simulink model "snb_bx"  (R2012b)
settings: Solver=FixedStepDiscrete  SolverMode=SingleTasking  StartTime=0.0  StopTime=10000  RelTol=1e-3
undefined symbols (not defined in the file): Down, pfb_coeff_gen_calc, Up, xlipgetpartsetting
libraries: xbsIndex_r4 x14917, casper_library_misc x20, casper_library_communications x8, xps_library x3, casper_library_delays x3
(part 48 of 96)

== system snb_bx/mix_dec_fir/dec_fir_async/fir_col_async3 ==
  dbus_in : Inport
  dbus_back_in : Inport  Port=2
  dv : Inport  Port=3
  adder_tree1 : Subsystem  AncestorBlock=casper_library_misc/adder_tree  mask(adder_tree){n_inputs=8, latency=3, adder_imp=Behavioral, first_stage_hdl=off}
      mask prompts: n_inputs "Number of Inputs"; latency "Add Latency"; adder_imp "Adder implementation"; first_stage_hdl "Use behavioural HDL for first stage of adders"
      mask help:
      | Sums all inputs using a tree of adds and delays.
      |
      | Number of inputs: The number of inputs to the block to be summed
      | Add latency: The number of clock cycles to perform one addition (affects timing)..
      | Adder implementation: choice of fabric or DSP48E core, or behavioral HDL
      | Use behavioural HDL for first stage of adders: Causes the first stage of adders to be absorbed into DSP blocks if multipliers precede them (Virtex 5). Overrides Adder implementation
      mask init:
      | adder_tree_init(gcb, ...
      |     'n_inputs', n_inputs, ...
      |     'latency', latency, ...
      |     'adder_imp', adder_imp, ...
      |     'first_stage_hdl', first_stage_hdl);
      settings: AttributesFormatString=latency 9
      mask Help: eval('xlWeb(''http://casper.berkeley.edu/wiki/Adder_tree'')')
      mask TypeOptions adder_imp: Behavioral | Fabric | DSP48
  adder_tree2 : Subsystem  AncestorBlock=casper_library_misc/adder_tree  mask(adder_tree){n_inputs=8, latency=3, adder_imp=Behavioral, first_stage_hdl=off}
      mask prompts: n_inputs "Number of Inputs"; latency "Add Latency"; adder_imp "Adder implementation"; first_stage_hdl "Use behavioural HDL for first stage of adders"
      mask help:
      | Sums all inputs using a tree of adds and delays.
      |
      | Number of inputs: The number of inputs to the block to be summed
      | Add latency: The number of clock cycles to perform one addition (affects timing)..
      | Adder implementation: choice of fabric or DSP48E core, or behavioral HDL
      | Use behavioural HDL for first stage of adders: Causes the first stage of adders to be absorbed into DSP blocks if multipliers precede them (Virtex 5). Overrides Adder implementation
      mask init:
      | adder_tree_init(gcb, ...
      |     'n_inputs', n_inputs, ...
      |     'latency', latency, ...
      |     'adder_imp', adder_imp, ...
      |     'first_stage_hdl', first_stage_hdl);
      settings: AttributesFormatString=latency 9
      mask Help: eval('xlWeb(''http://casper.berkeley.edu/wiki/Adder_tree'')')
      mask TypeOptions adder_imp: Behavioral | Fabric | DSP48
  c1 : xbsIndex_r4/Constant  const=1  gui_display_data_type=Fixed-point  arith_type=Signed (2's comp)  n_bits=16  bin_pt=14  preci_type=Single  exp_width=8  frac_width=24  explicit_period=on  period=1  equ=P=C  opselect=C  inp2=PCIN>>17  opr=+  inp1=P  carry=CIN  dbl_ovrd=off  block_type=constant
  c2 : xbsIndex_r4/Constant  const=1  gui_display_data_type=Fixed-point  arith_type=Signed (2's comp)  n_bits=16  bin_pt=14  preci_type=Single  exp_width=8  frac_width=24  explicit_period=on  period=1  equ=P=C  opselect=C  inp2=PCIN>>17  opr=+  inp1=P  carry=CIN  dbl_ovrd=off  block_type=constant
  fir_tap1 : Subsystem  AncestorBlock=casper_library_downconverter/fir_tap_async  mask(fir_tap_async){factor=0.028683, add_latency=3, mult_latency=2, coeff_bit_width=24, coeff_bin_pt=23, async=on, dbl=on}
      mask prompts: add_latency "Add latency"; mult_latency "Mult latency"; coeff_bit_width "Coefficient bit width"; coeff_bin_pt "Coefficient binary point"; async "Asynchronous ops"; dbl "Double tap"
      mask help: Multiplies input data with factor specified.
      mask init:
      | fir_tap_async_init(gcb);
      mask Help: eval('xlWeb(''http://casper.berkeley.edu/wiki/Fir_tap'')')
  fir_tap2 : Subsystem  AncestorBlock=casper_library_downconverter/fir_tap_async  mask(fir_tap_async){factor=0.026325, add_latency=3, mult_latency=2, coeff_bit_width=24, coeff_bin_pt=23, async=on, dbl=on}
      mask prompts: add_latency "Add latency"; mult_latency "Mult latency"; coeff_bit_width "Coefficient bit width"; coeff_bin_pt "Coefficient binary point"; async "Asynchronous ops"; dbl "Double tap"
      mask help: Multiplies input data with factor specified.
      mask init:
      | fir_tap_async_init(gcb);
      mask Help: eval('xlWeb(''http://casper.berkeley.edu/wiki/Fir_tap'')')
  fir_tap3 : Subsystem  AncestorBlock=casper_library_downconverter/fir_tap_async  mask(fir_tap_async){factor=0.023903, add_latency=3, mult_latency=2, coeff_bit_width=24, coeff_bin_pt=23, async=on, dbl=on}
      mask prompts: add_latency "Add latency"; mult_latency "Mult latency"; coeff_bit_width "Coefficient bit width"; coeff_bin_pt "Coefficient binary point"; async "Asynchronous ops"; dbl "Double tap"
      mask help: Multiplies input data with factor specified.
      mask init:
      | fir_tap_async_init(gcb);
      mask Help: eval('xlWeb(''http://casper.berkeley.edu/wiki/Fir_tap'')')
  fir_tap4 : Subsystem  AncestorBlock=casper_library_downconverter/fir_tap_async  mask(fir_tap_async){factor=0.021464, add_latency=3, mult_latency=2, coeff_bit_width=24, coeff_bin_pt=23, async=on, dbl=on}
      mask prompts: add_latency "Add latency"; mult_latency "Mult latency"; coeff_bit_width "Coefficient bit width"; coeff_bin_pt "Coefficient binary point"; async "Asynchronous ops"; dbl "Double tap"
      mask help: Multiplies input data with factor specified.
      mask init:
      | fir_tap_async_init(gcb);
      mask Help: eval('xlWeb(''http://casper.berkeley.edu/wiki/Fir_tap'')')
  fir_tap5 : Subsystem  AncestorBlock=casper_library_downconverter/fir_tap_async  mask(fir_tap_async){factor=0.01905, add_latency=3, mult_latency=2, coeff_bit_width=24, coeff_bin_pt=23, async=on, dbl=on}
      mask prompts: add_latency "Add latency"; mult_latency "Mult latency"; coeff_bit_width "Coefficient bit width"; coeff_bin_pt "Coefficient binary point"; async "Asynchronous ops"; dbl "Double tap"
      mask help: Multiplies input data with factor specified.
      mask init:
      | fir_tap_async_init(gcb);
      mask Help: eval('xlWeb(''http://casper.berkeley.edu/wiki/Fir_tap'')')
  fir_tap6 : Subsystem  AncestorBlock=casper_library_downconverter/fir_tap_async  mask(fir_tap_async){factor=0.016702, add_latency=3, mult_latency=2, coeff_bit_width=24, coeff_bin_pt=23, async=on, dbl=on}
      mask prompts: add_latency "Add latency"; mult_latency "Mult latency"; coeff_bit_width "Coefficient bit width"; coeff_bin_pt "Coefficient binary point"; async "Asynchronous ops"; dbl "Double tap"
      mask help: Multiplies input data with factor specified.
      mask init:
      | fir_tap_async_init(gcb);
      mask Help: eval('xlWeb(''http://casper.berkeley.edu/wiki/Fir_tap'')')
  fir_tap7 : Subsystem  AncestorBlock=casper_library_downconverter/fir_tap_async  mask(fir_tap_async){factor=0.014454, add_latency=3, mult_latency=2, coeff_bit_width=24, coeff_bin_pt=23, async=on, dbl=on}
      mask prompts: add_latency "Add latency"; mult_latency "Mult latency"; coeff_bit_width "Coefficient bit width"; coeff_bin_pt "Coefficient binary point"; async "Asynchronous ops"; dbl "Double tap"
      mask help: Multiplies input data with factor specified.
      mask init:
      | fir_tap_async_init(gcb);
      mask Help: eval('xlWeb(''http://casper.berkeley.edu/wiki/Fir_tap'')')
  fir_tap8 : Subsystem  AncestorBlock=casper_library_downconverter/fir_tap_async  mask(fir_tap_async){factor=0.012336, add_latency=3, mult_latency=2, coeff_bit_width=24, coeff_bin_pt=23, async=on, dbl=on}
      mask prompts: add_latency "Add latency"; mult_latency "Mult latency"; coeff_bit_width "Coefficient bit width"; coeff_bin_pt "Coefficient binary point"; async "Asynchronous ops"; dbl "Double tap"
      mask help: Multiplies input data with factor specified.
      mask init:
      | fir_tap_async_init(gcb);
      mask Help: eval('xlWeb(''http://casper.berkeley.edu/wiki/Fir_tap'')')
  inbus : Subsystem  AncestorBlock=casper_library_flow_control/bus_expand  mask(bus_expand){mode=divisions of equal size, outputNum=16, outputWidth=20, outputBinaryPt=18, outputArithmeticType=1, show_format=off, outputToWorkspace=off, variablePrefix=out, outputToModelAsWell=on}
      mask prompts: outputNum "Number of outputs:"; outputWidth "Output width:"; outputBinaryPt "Output binary point position:"; outputArithmeticType "Output arithmetic type (ufix=0, fix=1, bool=2):"; show_format "Print format string?"; outputToWorkspace "Output to workspace?"; variablePrefix "Variable name prefix:"; outputToModelAsWell "Output to model as well?"
      mask help:
      | Expands a 'bus' made using a bus_create or Xilinx
      | concat block.
      | The input will be divided into the specified number
      | of outputs with the specified arithmetic types.
      | Divisions are made from most significant bit.
      mask init: same as snb_bx/bus_expand10
      settings: AttributesFormatString=16 outputs
      mask TypeOptions mode: divisions of equal size | divisions of arbitrary size
      mask Callback mode: bus_expand_callback();
      mask Callback outputWidth: bus_expand_callback();
      mask Callback outputToWorkspace: bus_expand_callback();
  inbus_back : Subsystem  AncestorBlock=casper_library_flow_control/bus_expand  mask(bus_expand){mode=divisions of equal size, outputNum=16, outputWidth=20, outputBinaryPt=18, outputArithmeticType=1, show_format=off, outputToWorkspace=off, variablePrefix=out, outputToModelAsWell=on}
      mask prompts: outputNum "Number of outputs:"; outputWidth "Output width:"; outputBinaryPt "Output binary point position:"; outputArithmeticType "Output arithmetic type (ufix=0, fix=1, bool=2):"; show_format "Print format string?"; outputToWorkspace "Output to workspace?"; variablePrefix "Variable name prefix:"; outputToModelAsWell "Output to model as well?"
      mask help:
      | Expands a 'bus' made using a bus_create or Xilinx
      | concat block.
      | The input will be divided into the specified number
      | of outputs with the specified arithmetic types.
      | Divisions are made from most significant bit.
      mask init: same as snb_bx/bus_expand10
      settings: AttributesFormatString=16 outputs
      mask TypeOptions mode: divisions of equal size | divisions of arbitrary size
      mask Callback mode: bus_expand_callback();
      mask Callback outputWidth: bus_expand_callback();
      mask Callback outputToWorkspace: bus_expand_callback();
  outbus : Subsystem  AncestorBlock=casper_library_flow_control/bus_create  mask(bus_create){inputNum=16}
      mask prompts: inputNum "Number of inputs:"
      mask init:
      | bus_create_init(gcb,...
      |     'inputNum', inputNum);
  outbus_back : Subsystem  AncestorBlock=casper_library_flow_control/bus_create  mask(bus_create){inputNum=16}
      mask prompts: inputNum "Number of inputs:"
      mask init:
      | bus_create_init(gcb,...
      |     'inputNum', inputNum);
  term1 : Terminator
  term2 : Terminator
  dbus_out : Outport
  dbus_back_out : Outport  Port=2
  real_sum : Outport  Port=3
  imag_sum : Outport  Port=4
  wires:
  dbus_in/1 -> inbus/1(bus_in)
  dbus_back_in/1 -> inbus_back/1(bus_in)
  dv/1 -> [dv_in]
  [dv_in] -> fir_tap1/5(dv_in)
  inbus/1(msb_out16) -> fir_tap1/1(a)
  inbus/2(out15) -> fir_tap1/2(b)
  inbus_back/15(out2) -> fir_tap1/3(c)
  inbus_back/16(lsb_out1) -> fir_tap1/4(d)
  [dv_in] -> fir_tap2/5(dv_in)
  inbus/3(out14) -> fir_tap2/1(a)
  inbus/4(out13) -> fir_tap2/2(b)
  inbus_back/13(out4) -> fir_tap2/3(c)
  inbus_back/14(out3) -> fir_tap2/4(d)
  [dv_in] -> fir_tap3/5(dv_in)
  inbus/5(out12) -> fir_tap3/1(a)
  inbus/6(out11) -> fir_tap3/2(b)
  inbus_back/11(out6) -> fir_tap3/3(c)
  inbus_back/12(out5) -> fir_tap3/4(d)
  [dv_in] -> fir_tap4/5(dv_in)
  inbus/7(out10) -> fir_tap4/1(a)
  inbus/8(out9) -> fir_tap4/2(b)
  inbus_back/9(out8) -> fir_tap4/3(c)
  inbus_back/10(out7) -> fir_tap4/4(d)
  [dv_in] -> fir_tap5/5(dv_in)
  inbus/9(out8) -> fir_tap5/1(a)
  inbus/10(out7) -> fir_tap5/2(b)
  inbus_back/7(out10) -> fir_tap5/3(c)
  inbus_back/8(out9) -> fir_tap5/4(d)
  [dv_in] -> fir_tap6/5(dv_in)
  inbus/11(out6) -> fir_tap6/1(a)
  inbus/12(out5) -> fir_tap6/2(b)
  inbus_back/5(out12) -> fir_tap6/3(c)
  inbus_back/6(out11) -> fir_tap6/4(d)
  [dv_in] -> fir_tap7/5(dv_in)
  inbus/13(out4) -> fir_tap7/1(a)
  inbus/14(out3) -> fir_tap7/2(b)
  inbus_back/3(out14) -> fir_tap7/3(c)
  inbus_back/4(out13) -> fir_tap7/4(d)
  [dv_in] -> fir_tap8/5(dv_in)
  inbus/15(out2) -> fir_tap8/1(a)
  inbus/16(lsb_out1) -> fir_tap8/2(b)
  inbus_back/1(msb_out16) -> fir_tap8/3(c)
  inbus_back/2(out15) -> fir_tap8/4(d)
  outbus/1(bus_out) -> dbus_out/1
  outbus_back/1(bus_out) -> dbus_back_out/1
  fir_tap1/1(a_out) -> outbus/1(in1)
  fir_tap1/2(b_out) -> outbus/2(in2)
  fir_tap1/3(c_out) -> outbus_back/15(in15)
  fir_tap1/4(d_out) -> outbus_back/16(in16)
  fir_tap2/1(a_out) -> outbus/3(in3)
  fir_tap2/2(b_out) -> outbus/4(in4)
  fir_tap2/3(c_out) -> outbus_back/13(in13)
  fir_tap2/4(d_out) -> outbus_back/14(in14)
  fir_tap3/1(a_out) -> outbus/5(in5)
  fir_tap3/2(b_out) -> outbus/6(in6)
  fir_tap3/3(c_out) -> outbus_back/11(in11)
  fir_tap3/4(d_out) -> outbus_back/12(in12)
  fir_tap4/1(a_out) -> outbus/7(in7)
  fir_tap4/2(b_out) -> outbus/8(in8)
  fir_tap4/3(c_out) -> outbus_back/9(in9)
  fir_tap4/4(d_out) -> outbus_back/10(in10)
  fir_tap5/1(a_out) -> outbus/9(in9)
  fir_tap5/2(b_out) -> outbus/10(in10)
  fir_tap5/3(c_out) -> outbus_back/7(in7)
  fir_tap5/4(d_out) -> outbus_back/8(in8)
  fir_tap6/1(a_out) -> outbus/11(in11)
  fir_tap6/2(b_out) -> outbus/12(in12)
  fir_tap6/3(c_out) -> outbus_back/5(in5)
  fir_tap6/4(d_out) -> outbus_back/6(in6)
  fir_tap7/1(a_out) -> outbus/13(in13)
  fir_tap7/2(b_out) -> outbus/14(in14)
  fir_tap7/3(c_out) -> outbus_back/3(in3)
  fir_tap7/4(d_out) -> outbus_back/4(in4)
  fir_tap8/1(a_out) -> outbus/15(in15)
  fir_tap8/2(b_out) -> outbus/16(in16)
  fir_tap8/3(c_out) -> outbus_back/1(in1)
  fir_tap8/4(d_out) -> outbus_back/2(in2)
  adder_tree1/1(sync_out) -> term1/1
  adder_tree2/1(sync_out) -> term2/1
  c1/1 -> adder_tree1/1(sync)
  c2/1 -> adder_tree2/1(sync)
  adder_tree1/2(dout) -> real_sum/1
  adder_tree2/2(dout) -> imag_sum/1
  fir_tap1/5(real) -> adder_tree1/2(din1)
  fir_tap1/6(imag) -> adder_tree2/2(din1)
  fir_tap2/5(real) -> adder_tree1/3(din2)
  fir_tap2/6(imag) -> adder_tree2/3(din2)
  fir_tap3/5(real) -> adder_tree1/4(din3)
  fir_tap3/6(imag) -> adder_tree2/4(din3)
  fir_tap4/5(real) -> adder_tree1/5(din4)
  fir_tap4/6(imag) -> adder_tree2/5(din4)
  fir_tap5/5(real) -> adder_tree1/6(din5)
  fir_tap5/6(imag) -> adder_tree2/6(din5)
  fir_tap6/5(real) -> adder_tree1/7(din6)
  fir_tap6/6(imag) -> adder_tree2/7(din6)
  fir_tap7/5(real) -> adder_tree1/8(din7)
  fir_tap7/6(imag) -> adder_tree2/8(din7)
  fir_tap8/5(real) -> adder_tree1/9(din8)
  fir_tap8/6(imag) -> adder_tree2/9(din8)

== system snb_bx/mix_dec_fir/dec_fir_async/fir_col_async4 ==
  dbus_in : Inport
  dbus_back_in : Inport  Port=2
  dv : Inport  Port=3
  adder_tree1 : Subsystem  AncestorBlock=casper_library_misc/adder_tree  mask(adder_tree){n_inputs=8, latency=3, adder_imp=Behavioral, first_stage_hdl=off}
      mask prompts: n_inputs "Number of Inputs"; latency "Add Latency"; adder_imp "Adder implementation"; first_stage_hdl "Use behavioural HDL for first stage of adders"
      mask help:
      | Sums all inputs using a tree of adds and delays.
      |
      | Number of inputs: The number of inputs to the block to be summed
      | Add latency: The number of clock cycles to perform one addition (affects timing)..
      | Adder implementation: choice of fabric or DSP48E core, or behavioral HDL
      | Use behavioural HDL for first stage of adders: Causes the first stage of adders to be absorbed into DSP blocks if multipliers precede them (Virtex 5). Overrides Adder implementation
      mask init:
      | adder_tree_init(gcb, ...
      |     'n_inputs', n_inputs, ...
      |     'latency', latency, ...
      |     'adder_imp', adder_imp, ...
      |     'first_stage_hdl', first_stage_hdl);
      settings: AttributesFormatString=latency 9
      mask Help: eval('xlWeb(''http://casper.berkeley.edu/wiki/Adder_tree'')')
      mask TypeOptions adder_imp: Behavioral | Fabric | DSP48
  adder_tree2 : Subsystem  AncestorBlock=casper_library_misc/adder_tree  mask(adder_tree){n_inputs=8, latency=3, adder_imp=Behavioral, first_stage_hdl=off}
      mask prompts: n_inputs "Number of Inputs"; latency "Add Latency"; adder_imp "Adder implementation"; first_stage_hdl "Use behavioural HDL for first stage of adders"
      mask help:
      | Sums all inputs using a tree of adds and delays.
      |
      | Number of inputs: The number of inputs to the block to be summed
      | Add latency: The number of clock cycles to perform one addition (affects timing)..
      | Adder implementation: choice of fabric or DSP48E core, or behavioral HDL
      | Use behavioural HDL for first stage of adders: Causes the first stage of adders to be absorbed into DSP blocks if multipliers precede them (Virtex 5). Overrides Adder implementation
      mask init:
      | adder_tree_init(gcb, ...
      |     'n_inputs', n_inputs, ...
      |     'latency', latency, ...
      |     'adder_imp', adder_imp, ...
      |     'first_stage_hdl', first_stage_hdl);
      settings: AttributesFormatString=latency 9
      mask Help: eval('xlWeb(''http://casper.berkeley.edu/wiki/Adder_tree'')')
      mask TypeOptions adder_imp: Behavioral | Fabric | DSP48
  c1 : xbsIndex_r4/Constant  const=1  gui_display_data_type=Fixed-point  arith_type=Signed (2's comp)  n_bits=16  bin_pt=14  preci_type=Single  exp_width=8  frac_width=24  explicit_period=on  period=1  equ=P=C  opselect=C  inp2=PCIN>>17  opr=+  inp1=P  carry=CIN  dbl_ovrd=off  block_type=constant
  c2 : xbsIndex_r4/Constant  const=1  gui_display_data_type=Fixed-point  arith_type=Signed (2's comp)  n_bits=16  bin_pt=14  preci_type=Single  exp_width=8  frac_width=24  explicit_period=on  period=1  equ=P=C  opselect=C  inp2=PCIN>>17  opr=+  inp1=P  carry=CIN  dbl_ovrd=off  block_type=constant
  fir_tap1 : Subsystem  AncestorBlock=casper_library_downconverter/fir_tap_async  mask(fir_tap_async){factor=0.040055, add_latency=3, mult_latency=2, coeff_bit_width=24, coeff_bin_pt=23, async=on, dbl=on}
      mask prompts: add_latency "Add latency"; mult_latency "Mult latency"; coeff_bit_width "Coefficient bit width"; coeff_bin_pt "Coefficient binary point"; async "Asynchronous ops"; dbl "Double tap"
      mask help: Multiplies input data with factor specified.
      mask init:
      | fir_tap_async_init(gcb);
      mask Help: eval('xlWeb(''http://casper.berkeley.edu/wiki/Fir_tap'')')
  fir_tap2 : Subsystem  AncestorBlock=casper_library_downconverter/fir_tap_async  mask(fir_tap_async){factor=0.039693, add_latency=3, mult_latency=2, coeff_bit_width=24, coeff_bin_pt=23, async=on, dbl=on}
      mask prompts: add_latency "Add latency"; mult_latency "Mult latency"; coeff_bit_width "Coefficient bit width"; coeff_bin_pt "Coefficient binary point"; async "Asynchronous ops"; dbl "Double tap"
      mask help: Multiplies input data with factor specified.
      mask init:
      | fir_tap_async_init(gcb);
      mask Help: eval('xlWeb(''http://casper.berkeley.edu/wiki/Fir_tap'')')
  fir_tap3 : Subsystem  AncestorBlock=casper_library_downconverter/fir_tap_async  mask(fir_tap_async){factor=0.038977, add_latency=3, mult_latency=2, coeff_bit_width=24, coeff_bin_pt=23, async=on, dbl=on}
      mask prompts: add_latency "Add latency"; mult_latency "Mult latency"; coeff_bit_width "Coefficient bit width"; coeff_bin_pt "Coefficient binary point"; async "Asynchronous ops"; dbl "Double tap"
      mask help: Multiplies input data with factor specified.
      mask init:
      | fir_tap_async_init(gcb);
      mask Help: eval('xlWeb(''http://casper.berkeley.edu/wiki/Fir_tap'')')
  fir_tap4 : Subsystem  AncestorBlock=casper_library_downconverter/fir_tap_async  mask(fir_tap_async){factor=0.037924, add_latency=3, mult_latency=2, coeff_bit_width=24, coeff_bin_pt=23, async=on, dbl=on}
      mask prompts: add_latency "Add latency"; mult_latency "Mult latency"; coeff_bit_width "Coefficient bit width"; coeff_bin_pt "Coefficient binary point"; async "Asynchronous ops"; dbl "Double tap"
      mask help: Multiplies input data with factor specified.
      mask init:
      | fir_tap_async_init(gcb);
      mask Help: eval('xlWeb(''http://casper.berkeley.edu/wiki/Fir_tap'')')
  fir_tap5 : Subsystem  AncestorBlock=casper_library_downconverter/fir_tap_async  mask(fir_tap_async){factor=0.036558, add_latency=3, mult_latency=2, coeff_bit_width=24, coeff_bin_pt=23, async=on, dbl=on}
      mask prompts: add_latency "Add latency"; mult_latency "Mult latency"; coeff_bit_width "Coefficient bit width"; coeff_bin_pt "Coefficient binary point"; async "Asynchronous ops"; dbl "Double tap"
      mask help: Multiplies input data with factor specified.
      mask init:
      | fir_tap_async_init(gcb);
      mask Help: eval('xlWeb(''http://casper.berkeley.edu/wiki/Fir_tap'')')
  fir_tap6 : Subsystem  AncestorBlock=casper_library_downconverter/fir_tap_async  mask(fir_tap_async){factor=0.034912, add_latency=3, mult_latency=2, coeff_bit_width=24, coeff_bin_pt=23, async=on, dbl=on}
      mask prompts: add_latency "Add latency"; mult_latency "Mult latency"; coeff_bit_width "Coefficient bit width"; coeff_bin_pt "Coefficient binary point"; async "Asynchronous ops"; dbl "Double tap"
      mask help: Multiplies input data with factor specified.
      mask init:
      | fir_tap_async_init(gcb);
      mask Help: eval('xlWeb(''http://casper.berkeley.edu/wiki/Fir_tap'')')
  fir_tap7 : Subsystem  AncestorBlock=casper_library_downconverter/fir_tap_async  mask(fir_tap_async){factor=0.033023, add_latency=3, mult_latency=2, coeff_bit_width=24, coeff_bin_pt=23, async=on, dbl=on}
      mask prompts: add_latency "Add latency"; mult_latency "Mult latency"; coeff_bit_width "Coefficient bit width"; coeff_bin_pt "Coefficient binary point"; async "Asynchronous ops"; dbl "Double tap"
      mask help: Multiplies input data with factor specified.
      mask init:
      | fir_tap_async_init(gcb);
      mask Help: eval('xlWeb(''http://casper.berkeley.edu/wiki/Fir_tap'')')
  fir_tap8 : Subsystem  AncestorBlock=casper_library_downconverter/fir_tap_async  mask(fir_tap_async){factor=0.030931, add_latency=3, mult_latency=2, coeff_bit_width=24, coeff_bin_pt=23, async=on, dbl=on}
      mask prompts: add_latency "Add latency"; mult_latency "Mult latency"; coeff_bit_width "Coefficient bit width"; coeff_bin_pt "Coefficient binary point"; async "Asynchronous ops"; dbl "Double tap"
      mask help: Multiplies input data with factor specified.
      mask init:
      | fir_tap_async_init(gcb);
      mask Help: eval('xlWeb(''http://casper.berkeley.edu/wiki/Fir_tap'')')
  inbus : Subsystem  AncestorBlock=casper_library_flow_control/bus_expand  mask(bus_expand){mode=divisions of equal size, outputNum=16, outputWidth=20, outputBinaryPt=18, outputArithmeticType=1, show_format=off, outputToWorkspace=off, variablePrefix=out, outputToModelAsWell=on}
      mask prompts: outputNum "Number of outputs:"; outputWidth "Output width:"; outputBinaryPt "Output binary point position:"; outputArithmeticType "Output arithmetic type (ufix=0, fix=1, bool=2):"; show_format "Print format string?"; outputToWorkspace "Output to workspace?"; variablePrefix "Variable name prefix:"; outputToModelAsWell "Output to model as well?"
      mask help:
      | Expands a 'bus' made using a bus_create or Xilinx
      | concat block.
      | The input will be divided into the specified number
      | of outputs with the specified arithmetic types.
      | Divisions are made from most significant bit.
      mask init: same as snb_bx/bus_expand10
      settings: AttributesFormatString=16 outputs
      mask TypeOptions mode: divisions of equal size | divisions of arbitrary size
      mask Callback mode: bus_expand_callback();
      mask Callback outputWidth: bus_expand_callback();
      mask Callback outputToWorkspace: bus_expand_callback();
  inbus_back : Subsystem  AncestorBlock=casper_library_flow_control/bus_expand  mask(bus_expand){mode=divisions of equal size, outputNum=16, outputWidth=20, outputBinaryPt=18, outputArithmeticType=1, show_format=off, outputToWorkspace=off, variablePrefix=out, outputToModelAsWell=on}
      mask prompts: outputNum "Number of outputs:"; outputWidth "Output width:"; outputBinaryPt "Output binary point position:"; outputArithmeticType "Output arithmetic type (ufix=0, fix=1, bool=2):"; show_format "Print format string?"; outputToWorkspace "Output to workspace?"; variablePrefix "Variable name prefix:"; outputToModelAsWell "Output to model as well?"
      mask help:
      | Expands a 'bus' made using a bus_create or Xilinx
      | concat block.
      | The input will be divided into the specified number
      | of outputs with the specified arithmetic types.
      | Divisions are made from most significant bit.
      mask init: same as snb_bx/bus_expand10
      settings: AttributesFormatString=16 outputs
      mask TypeOptions mode: divisions of equal size | divisions of arbitrary size
      mask Callback mode: bus_expand_callback();
      mask Callback outputWidth: bus_expand_callback();
      mask Callback outputToWorkspace: bus_expand_callback();
  outbus : Subsystem  AncestorBlock=casper_library_flow_control/bus_create  mask(bus_create){inputNum=16}
      mask prompts: inputNum "Number of inputs:"
      mask init:
      | bus_create_init(gcb,...
      |     'inputNum', inputNum);
  outbus_back : Subsystem  AncestorBlock=casper_library_flow_control/bus_create  mask(bus_create){inputNum=16}
      mask prompts: inputNum "Number of inputs:"
      mask init:
      | bus_create_init(gcb,...
      |     'inputNum', inputNum);
  term1 : Terminator
  term2 : Terminator
  dbus_out : Outport
  dbus_back_out : Outport  Port=2
  real_sum : Outport  Port=3
  imag_sum : Outport  Port=4
  wires:
  dbus_in/1 -> inbus/1(bus_in)
  dbus_back_in/1 -> inbus_back/1(bus_in)
  dv/1 -> [dv_in]
  [dv_in] -> fir_tap1/5(dv_in)
  inbus/1(msb_out16) -> fir_tap1/1(a)
  inbus/2(out15) -> fir_tap1/2(b)
  inbus_back/15(out2) -> fir_tap1/3(c)
  inbus_back/16(lsb_out1) -> fir_tap1/4(d)
  [dv_in] -> fir_tap2/5(dv_in)
  inbus/3(out14) -> fir_tap2/1(a)
  inbus/4(out13) -> fir_tap2/2(b)
  inbus_back/13(out4) -> fir_tap2/3(c)
  inbus_back/14(out3) -> fir_tap2/4(d)
  [dv_in] -> fir_tap3/5(dv_in)
  inbus/5(out12) -> fir_tap3/1(a)
  inbus/6(out11) -> fir_tap3/2(b)
  inbus_back/11(out6) -> fir_tap3/3(c)
  inbus_back/12(out5) -> fir_tap3/4(d)
  [dv_in] -> fir_tap4/5(dv_in)
  inbus/7(out10) -> fir_tap4/1(a)
  inbus/8(out9) -> fir_tap4/2(b)
  inbus_back/9(out8) -> fir_tap4/3(c)
  inbus_back/10(out7) -> fir_tap4/4(d)
  [dv_in] -> fir_tap5/5(dv_in)
  inbus/9(out8) -> fir_tap5/1(a)
  inbus/10(out7) -> fir_tap5/2(b)
  inbus_back/7(out10) -> fir_tap5/3(c)
  inbus_back/8(out9) -> fir_tap5/4(d)
  [dv_in] -> fir_tap6/5(dv_in)
  inbus/11(out6) -> fir_tap6/1(a)
  inbus/12(out5) -> fir_tap6/2(b)
  inbus_back/5(out12) -> fir_tap6/3(c)
  inbus_back/6(out11) -> fir_tap6/4(d)
  [dv_in] -> fir_tap7/5(dv_in)
  inbus/13(out4) -> fir_tap7/1(a)
  inbus/14(out3) -> fir_tap7/2(b)
  inbus_back/3(out14) -> fir_tap7/3(c)
  inbus_back/4(out13) -> fir_tap7/4(d)
  [dv_in] -> fir_tap8/5(dv_in)
  inbus/15(out2) -> fir_tap8/1(a)
  inbus/16(lsb_out1) -> fir_tap8/2(b)
  inbus_back/1(msb_out16) -> fir_tap8/3(c)
  inbus_back/2(out15) -> fir_tap8/4(d)
  outbus/1(bus_out) -> dbus_out/1
  outbus_back/1(bus_out) -> dbus_back_out/1
  fir_tap1/1(a_out) -> outbus/1(in1)
  fir_tap1/2(b_out) -> outbus/2(in2)
  fir_tap1/3(c_out) -> outbus_back/15(in15)
  fir_tap1/4(d_out) -> outbus_back/16(in16)
  fir_tap2/1(a_out) -> outbus/3(in3)
  fir_tap2/2(b_out) -> outbus/4(in4)
  fir_tap2/3(c_out) -> outbus_back/13(in13)
  fir_tap2/4(d_out) -> outbus_back/14(in14)
  fir_tap3/1(a_out) -> outbus/5(in5)
  fir_tap3/2(b_out) -> outbus/6(in6)
  fir_tap3/3(c_out) -> outbus_back/11(in11)
  fir_tap3/4(d_out) -> outbus_back/12(in12)
  fir_tap4/1(a_out) -> outbus/7(in7)
  fir_tap4/2(b_out) -> outbus/8(in8)
  fir_tap4/3(c_out) -> outbus_back/9(in9)
  fir_tap4/4(d_out) -> outbus_back/10(in10)
  fir_tap5/1(a_out) -> outbus/9(in9)
  fir_tap5/2(b_out) -> outbus/10(in10)
  fir_tap5/3(c_out) -> outbus_back/7(in7)
  fir_tap5/4(d_out) -> outbus_back/8(in8)
  fir_tap6/1(a_out) -> outbus/11(in11)
  fir_tap6/2(b_out) -> outbus/12(in12)
  fir_tap6/3(c_out) -> outbus_back/5(in5)
  fir_tap6/4(d_out) -> outbus_back/6(in6)
  fir_tap7/1(a_out) -> outbus/13(in13)
  fir_tap7/2(b_out) -> outbus/14(in14)
  fir_tap7/3(c_out) -> outbus_back/3(in3)
  fir_tap7/4(d_out) -> outbus_back/4(in4)
  fir_tap8/1(a_out) -> outbus/15(in15)
  fir_tap8/2(b_out) -> outbus/16(in16)
  fir_tap8/3(c_out) -> outbus_back/1(in1)
  fir_tap8/4(d_out) -> outbus_back/2(in2)
  adder_tree1/1(sync_out) -> term1/1
  adder_tree2/1(sync_out) -> term2/1
  c1/1 -> adder_tree1/1(sync)
  c2/1 -> adder_tree2/1(sync)
  adder_tree1/2(dout) -> real_sum/1
  adder_tree2/2(dout) -> imag_sum/1
  fir_tap1/5(real) -> adder_tree1/2(din1)
  fir_tap1/6(imag) -> adder_tree2/2(din1)
  fir_tap2/5(real) -> adder_tree1/3(din2)
  fir_tap2/6(imag) -> adder_tree2/3(din2)
  fir_tap3/5(real) -> adder_tree1/4(din3)
  fir_tap3/6(imag) -> adder_tree2/4(din3)
  fir_tap4/5(real) -> adder_tree1/5(din4)
  fir_tap4/6(imag) -> adder_tree2/5(din4)
  fir_tap5/5(real) -> adder_tree1/6(din5)
  fir_tap5/6(imag) -> adder_tree2/6(din5)
  fir_tap6/5(real) -> adder_tree1/7(din6)
  fir_tap6/6(imag) -> adder_tree2/7(din6)
  fir_tap7/5(real) -> adder_tree1/8(din7)
  fir_tap7/6(imag) -> adder_tree2/8(din7)
  fir_tap8/5(real) -> adder_tree1/9(din8)
  fir_tap8/6(imag) -> adder_tree2/9(din8)

== system snb_bx/mix_dec_fir/dec_fir_async/imag_sum ==
  sync : Inport
  din1 : Inport  Port=2
  din2 : Inport  Port=3
  din3 : Inport  Port=4
  din4 : Inport  Port=5
  addr1 : xbsIndex_r4/AddSub  mode=Addition  use_carryin=off  use_carryout=off  en=off  latency=3  precision=Full  arith_type=Unsigned  n_bits=16  bin_pt=14  quantization=Truncate  overflow=Wrap  dbl_ovrd=off  use_behavioral_HDL=on  hw_selection=Fabric  pipelined=on  use_rpm=on  block_type=addsub
  addr2 : xbsIndex_r4/AddSub  mode=Addition  use_carryin=off  use_carryout=off  en=off  latency=3  precision=Full  arith_type=Unsigned  n_bits=16  bin_pt=14  quantization=Truncate  overflow=Wrap  dbl_ovrd=off  use_behavioral_HDL=on  hw_selection=Fabric  pipelined=on  use_rpm=on  block_type=addsub
  addr3 : xbsIndex_r4/AddSub  mode=Addition  use_carryin=off  use_carryout=off  en=off  latency=3  precision=Full  arith_type=Unsigned  n_bits=16  bin_pt=14  quantization=Truncate  overflow=Wrap  dbl_ovrd=off  use_behavioral_HDL=on  hw_selection=Fabric  pipelined=on  use_rpm=on  block_type=addsub
  sync_delay : xbsIndex_r4/Delay  rst=off  infoeditControl=Selection of Reset will increase slice count due to use of real FFs and instead of SRLs  en=off  latency=6  dbl_ovrd=off  reg_retiming=on  block_type=delay
      settings: block_version=11.4
  sync_out : Outport
  dout : Outport  Port=2
  wires:
  sync/1 -> sync_delay/1
  sync_delay/1 -> sync_out/1
  din1/1 -> addr1/1
  din2/1 -> addr1/2
  din3/1 -> addr2/1
  din4/1 -> addr2/2
  addr1/1 -> addr3/1
  addr2/1 -> addr3/2
  addr3/1 -> dout/1

== system snb_bx/mix_dec_fir/dec_fir_async/real_sum ==
  sync : Inport
  din1 : Inport  Port=2
  din2 : Inport  Port=3
  din3 : Inport  Port=4
  din4 : Inport  Port=5
  addr1 : xbsIndex_r4/AddSub  mode=Addition  use_carryin=off  use_carryout=off  en=off  latency=3  precision=Full  arith_type=Unsigned  n_bits=16  bin_pt=14  quantization=Truncate  overflow=Wrap  dbl_ovrd=off  use_behavioral_HDL=on  hw_selection=Fabric  pipelined=on  use_rpm=on  block_type=addsub
  addr2 : xbsIndex_r4/AddSub  mode=Addition  use_carryin=off  use_carryout=off  en=off  latency=3  precision=Full  arith_type=Unsigned  n_bits=16  bin_pt=14  quantization=Truncate  overflow=Wrap  dbl_ovrd=off  use_behavioral_HDL=on  hw_selection=Fabric  pipelined=on  use_rpm=on  block_type=addsub
  addr3 : xbsIndex_r4/AddSub  mode=Addition  use_carryin=off  use_carryout=off  en=off  latency=3  precision=Full  arith_type=Unsigned  n_bits=16  bin_pt=14  quantization=Truncate  overflow=Wrap  dbl_ovrd=off  use_behavioral_HDL=on  hw_selection=Fabric  pipelined=on  use_rpm=on  block_type=addsub
  sync_delay : xbsIndex_r4/Delay  rst=off  infoeditControl=Selection of Reset will increase slice count due to use of real FFs and instead of SRLs  en=off  latency=6  dbl_ovrd=off  reg_retiming=on  block_type=delay
      settings: block_version=11.4
  sync_out : Outport
  dout : Outport  Port=2
  wires:
  sync/1 -> sync_delay/1
  sync_delay/1 -> sync_out/1
  din1/1 -> addr1/1
  din2/1 -> addr1/2
  din3/1 -> addr2/1
  din4/1 -> addr2/2
  addr1/1 -> addr3/1
  addr2/1 -> addr3/2
  addr3/1 -> dout/1

== system snb_bx/mix_dec_fir/dec_fir_async1/fir_col_async1 ==
  dbus_in : Inport
  dbus_back_in : Inport  Port=2
  dv : Inport  Port=3
  adder_tree1 : Subsystem  AncestorBlock=casper_library_misc/adder_tree  mask(adder_tree){n_inputs=8, latency=3, adder_imp=Behavioral, first_stage_hdl=off}
      mask prompts: n_inputs "Number of Inputs"; latency "Add Latency"; adder_imp "Adder implementation"; first_stage_hdl "Use behavioural HDL for first stage of adders"
      mask help:
      | Sums all inputs using a tree of adds and delays.
      |
      | Number of inputs: The number of inputs to the block to be summed
      | Add latency: The number of clock cycles to perform one addition (affects timing)..
      | Adder implementation: choice of fabric or DSP48E core, or behavioral HDL
      | Use behavioural HDL for first stage of adders: Causes the first stage of adders to be absorbed into DSP blocks if multipliers precede them (Virtex 5). Overrides Adder implementation
      mask init:
      | adder_tree_init(gcb, ...
      |     'n_inputs', n_inputs, ...
      |     'latency', latency, ...
      |     'adder_imp', adder_imp, ...
      |     'first_stage_hdl', first_stage_hdl);
      settings: AttributesFormatString=latency 9
      mask Help: eval('xlWeb(''http://casper.berkeley.edu/wiki/Adder_tree'')')
      mask TypeOptions adder_imp: Behavioral | Fabric | DSP48
  adder_tree2 : Subsystem  AncestorBlock=casper_library_misc/adder_tree  mask(adder_tree){n_inputs=8, latency=3, adder_imp=Behavioral, first_stage_hdl=off}
      mask prompts: n_inputs "Number of Inputs"; latency "Add Latency"; adder_imp "Adder implementation"; first_stage_hdl "Use behavioural HDL for first stage of adders"
      mask help:
      | Sums all inputs using a tree of adds and delays.
      |
      | Number of inputs: The number of inputs to the block to be summed
      | Add latency: The number of clock cycles to perform one addition (affects timing)..
      | Adder implementation: choice of fabric or DSP48E core, or behavioral HDL
      | Use behavioural HDL for first stage of adders: Causes the first stage of adders to be absorbed into DSP blocks if multipliers precede them (Virtex 5). Overrides Adder implementation
      mask init:
      | adder_tree_init(gcb, ...
      |     'n_inputs', n_inputs, ...
      |     'latency', latency, ...
      |     'adder_imp', adder_imp, ...
      |     'first_stage_hdl', first_stage_hdl);
      settings: AttributesFormatString=latency 9
      mask Help: eval('xlWeb(''http://casper.berkeley.edu/wiki/Adder_tree'')')
      mask TypeOptions adder_imp: Behavioral | Fabric | DSP48
  c1 : xbsIndex_r4/Constant  const=1  gui_display_data_type=Fixed-point  arith_type=Signed (2's comp)  n_bits=16  bin_pt=14  preci_type=Single  exp_width=8  frac_width=24  explicit_period=on  period=1  equ=P=C  opselect=C  inp2=PCIN>>17  opr=+  inp1=P  carry=CIN  dbl_ovrd=off  block_type=constant
  c2 : xbsIndex_r4/Constant  const=1  gui_display_data_type=Fixed-point  arith_type=Signed (2's comp)  n_bits=16  bin_pt=14  preci_type=Single  exp_width=8  frac_width=24  explicit_period=on  period=1  equ=P=C  opselect=C  inp2=PCIN>>17  opr=+  inp1=P  carry=CIN  dbl_ovrd=off  block_type=constant
  fir_tap1 : Subsystem  AncestorBlock=casper_library_downconverter/fir_tap_async  mask(fir_tap_async){factor=0.0011249, add_latency=3, mult_latency=2, coeff_bit_width=24, coeff_bin_pt=23, async=on, dbl=on}
      mask prompts: add_latency "Add latency"; mult_latency "Mult latency"; coeff_bit_width "Coefficient bit width"; coeff_bin_pt "Coefficient binary point"; async "Asynchronous ops"; dbl "Double tap"
      mask help: Multiplies input data with factor specified.
      mask init:
      | fir_tap_async_init(gcb);
      mask Help: eval('xlWeb(''http://casper.berkeley.edu/wiki/Fir_tap'')')
  fir_tap2 : Subsystem  AncestorBlock=casper_library_downconverter/fir_tap_async  mask(fir_tap_async){factor=0.0006933, add_latency=3, mult_latency=2, coeff_bit_width=24, coeff_bin_pt=23, async=on, dbl=on}
      mask prompts: add_latency "Add latency"; mult_latency "Mult latency"; coeff_bit_width "Coefficient bit width"; coeff_bin_pt "Coefficient binary point"; async "Asynchronous ops"; dbl "Double tap"
      mask help: Multiplies input data with factor specified.
      mask init:
      | fir_tap_async_init(gcb);
      mask Help: eval('xlWeb(''http://casper.berkeley.edu/wiki/Fir_tap'')')
  fir_tap3 : Subsystem  AncestorBlock=casper_library_downconverter/fir_tap_async  mask(fir_tap_async){factor=0.00037455, add_latency=3, mult_latency=2, coeff_bit_width=24, coeff_bin_pt=23, async=on, dbl=on}
      mask prompts: add_latency "Add latency"; mult_latency "Mult latency"; coeff_bit_width "Coefficient bit width"; coeff_bin_pt "Coefficient binary point"; async "Asynchronous ops"; dbl "Double tap"
      mask help: Multiplies input data with factor specified.
      mask init:
      | fir_tap_async_init(gcb);
      mask Help: eval('xlWeb(''http://casper.berkeley.edu/wiki/Fir_tap'')')
  fir_tap4 : Subsystem  AncestorBlock=casper_library_downconverter/fir_tap_async  mask(fir_tap_async){factor=0.00015055, add_latency=3, mult_latency=2, coeff_bit_width=24, coeff_bin_pt=23, async=on, dbl=on}
      mask prompts: add_latency "Add latency"; mult_latency "Mult latency"; coeff_bit_width "Coefficient bit width"; coeff_bin_pt "Coefficient binary point"; async "Asynchronous ops"; dbl "Double tap"
      mask help: Multiplies input data with factor specified.
      mask init:
      | fir_tap_async_init(gcb);
      mask Help: eval('xlWeb(''http://casper.berkeley.edu/wiki/Fir_tap'')')
  fir_tap5 : Subsystem  AncestorBlock=casper_library_downconverter/fir_tap_async  mask(fir_tap_async){factor=3.7598e-06, add_latency=3, mult_latency=2, coeff_bit_width=24, coeff_bin_pt=23, async=on, dbl=on}
      mask prompts: add_latency "Add latency"; mult_latency "Mult latency"; coeff_bit_width "Coefficient bit width"; coeff_bin_pt "Coefficient binary point"; async "Asynchronous ops"; dbl "Double tap"
      mask help: Multiplies input data with factor specified.
      mask init:
      | fir_tap_async_init(gcb);
      mask Help: eval('xlWeb(''http://casper.berkeley.edu/wiki/Fir_tap'')')
  fir_tap6 : Subsystem  AncestorBlock=casper_library_downconverter/fir_tap_async  mask(fir_tap_async){factor=-8.2327e-05, add_latency=3, mult_latency=2, coeff_bit_width=24, coeff_bin_pt=23, async=on, dbl=on}
      mask prompts: add_latency "Add latency"; mult_latency "Mult latency"; coeff_bit_width "Coefficient bit width"; coeff_bin_pt "Coefficient binary point"; async "Asynchronous ops"; dbl "Double tap"
      mask help: Multiplies input data with factor specified.
      mask init:
      | fir_tap_async_init(gcb);
      mask Help: eval('xlWeb(''http://casper.berkeley.edu/wiki/Fir_tap'')')
  fir_tap7 : Subsystem  AncestorBlock=casper_library_downconverter/fir_tap_async  mask(fir_tap_async){factor=-0.00012272, add_latency=3, mult_latency=2, coeff_bit_width=24, coeff_bin_pt=23, async=on, dbl=on}
      mask prompts: add_latency "Add latency"; mult_latency "Mult latency"; coeff_bit_width "Coefficient bit width"; coeff_bin_pt "Coefficient binary point"; async "Asynchronous ops"; dbl "Double tap"
      mask help: Multiplies input data with factor specified.
      mask init:
      | fir_tap_async_init(gcb);
      mask Help: eval('xlWeb(''http://casper.berkeley.edu/wiki/Fir_tap'')')
  fir_tap8 : Subsystem  AncestorBlock=casper_library_downconverter/fir_tap_async  mask(fir_tap_async){factor=-0.00027065, add_latency=3, mult_latency=2, coeff_bit_width=24, coeff_bin_pt=23, async=on, dbl=on}
      mask prompts: add_latency "Add latency"; mult_latency "Mult latency"; coeff_bit_width "Coefficient bit width"; coeff_bin_pt "Coefficient binary point"; async "Asynchronous ops"; dbl "Double tap"
      mask help: Multiplies input data with factor specified.
      mask init:
      | fir_tap_async_init(gcb);
      mask Help: eval('xlWeb(''http://casper.berkeley.edu/wiki/Fir_tap'')')
  inbus : Subsystem  AncestorBlock=casper_library_flow_control/bus_expand  mask(bus_expand){mode=divisions of equal size, outputNum=16, outputWidth=20, outputBinaryPt=18, outputArithmeticType=1, show_format=off, outputToWorkspace=off, variablePrefix=out, outputToModelAsWell=on}
      mask prompts: outputNum "Number of outputs:"; outputWidth "Output width:"; outputBinaryPt "Output binary point position:"; outputArithmeticType "Output arithmetic type (ufix=0, fix=1, bool=2):"; show_format "Print format string?"; outputToWorkspace "Output to workspace?"; variablePrefix "Variable name prefix:"; outputToModelAsWell "Output to model as well?"
      mask help:
      | Expands a 'bus' made using a bus_create or Xilinx
      | concat block.
      | The input will be divided into the specified number
      | of outputs with the specified arithmetic types.
      | Divisions are made from most significant bit.
      mask init: same as snb_bx/bus_expand10
      settings: AttributesFormatString=16 outputs
      mask TypeOptions mode: divisions of equal size | divisions of arbitrary size
      mask Callback mode: bus_expand_callback();
      mask Callback outputWidth: bus_expand_callback();
      mask Callback outputToWorkspace: bus_expand_callback();
  inbus_back : Subsystem  AncestorBlock=casper_library_flow_control/bus_expand  mask(bus_expand){mode=divisions of equal size, outputNum=16, outputWidth=20, outputBinaryPt=18, outputArithmeticType=1, show_format=off, outputToWorkspace=off, variablePrefix=out, outputToModelAsWell=on}
      mask prompts: outputNum "Number of outputs:"; outputWidth "Output width:"; outputBinaryPt "Output binary point position:"; outputArithmeticType "Output arithmetic type (ufix=0, fix=1, bool=2):"; show_format "Print format string?"; outputToWorkspace "Output to workspace?"; variablePrefix "Variable name prefix:"; outputToModelAsWell "Output to model as well?"
      mask help:
      | Expands a 'bus' made using a bus_create or Xilinx
      | concat block.
      | The input will be divided into the specified number
      | of outputs with the specified arithmetic types.
      | Divisions are made from most significant bit.
      mask init: same as snb_bx/bus_expand10
      settings: AttributesFormatString=16 outputs
      mask TypeOptions mode: divisions of equal size | divisions of arbitrary size
      mask Callback mode: bus_expand_callback();
      mask Callback outputWidth: bus_expand_callback();
      mask Callback outputToWorkspace: bus_expand_callback();
  outbus : Subsystem  AncestorBlock=casper_library_flow_control/bus_create  mask(bus_create){inputNum=16}
      mask prompts: inputNum "Number of inputs:"
      mask init:
      | bus_create_init(gcb,...
      |     'inputNum', inputNum);
  outbus_back : Subsystem  AncestorBlock=casper_library_flow_control/bus_create  mask(bus_create){inputNum=16}
      mask prompts: inputNum "Number of inputs:"
      mask init:
      | bus_create_init(gcb,...
      |     'inputNum', inputNum);
  term1 : Terminator
  term2 : Terminator
  dbus_out : Outport
  dbus_back_out : Outport  Port=2
  real_sum : Outport  Port=3
  imag_sum : Outport  Port=4
  wires:
  dbus_in/1 -> inbus/1(bus_in)
  dbus_back_in/1 -> inbus_back/1(bus_in)
  dv/1 -> [dv_in]
  [dv_in] -> fir_tap1/5(dv_in)
  inbus/1(msb_out16) -> fir_tap1/1(a)
  inbus/2(out15) -> fir_tap1/2(b)
  inbus_back/15(out2) -> fir_tap1/3(c)
  inbus_back/16(lsb_out1) -> fir_tap1/4(d)
  [dv_in] -> fir_tap2/5(dv_in)
  inbus/3(out14) -> fir_tap2/1(a)
  inbus/4(out13) -> fir_tap2/2(b)
  inbus_back/13(out4) -> fir_tap2/3(c)
  inbus_back/14(out3) -> fir_tap2/4(d)
  [dv_in] -> fir_tap3/5(dv_in)
  inbus/5(out12) -> fir_tap3/1(a)
  inbus/6(out11) -> fir_tap3/2(b)
  inbus_back/11(out6) -> fir_tap3/3(c)
  inbus_back/12(out5) -> fir_tap3/4(d)
  [dv_in] -> fir_tap4/5(dv_in)
  inbus/7(out10) -> fir_tap4/1(a)
  inbus/8(out9) -> fir_tap4/2(b)
  inbus_back/9(out8) -> fir_tap4/3(c)
  inbus_back/10(out7) -> fir_tap4/4(d)
  [dv_in] -> fir_tap5/5(dv_in)
  inbus/9(out8) -> fir_tap5/1(a)
  inbus/10(out7) -> fir_tap5/2(b)
  inbus_back/7(out10) -> fir_tap5/3(c)
  inbus_back/8(out9) -> fir_tap5/4(d)
  [dv_in] -> fir_tap6/5(dv_in)
  inbus/11(out6) -> fir_tap6/1(a)
  inbus/12(out5) -> fir_tap6/2(b)
  inbus_back/5(out12) -> fir_tap6/3(c)
  inbus_back/6(out11) -> fir_tap6/4(d)
  [dv_in] -> fir_tap7/5(dv_in)
  inbus/13(out4) -> fir_tap7/1(a)
  inbus/14(out3) -> fir_tap7/2(b)
  inbus_back/3(out14) -> fir_tap7/3(c)
  inbus_back/4(out13) -> fir_tap7/4(d)
  [dv_in] -> fir_tap8/5(dv_in)
  inbus/15(out2) -> fir_tap8/1(a)
  inbus/16(lsb_out1) -> fir_tap8/2(b)
  inbus_back/1(msb_out16) -> fir_tap8/3(c)
  inbus_back/2(out15) -> fir_tap8/4(d)
  outbus/1(bus_out) -> dbus_out/1
  outbus_back/1(bus_out) -> dbus_back_out/1
  fir_tap1/1(a_out) -> outbus/1(in1)
  fir_tap1/2(b_out) -> outbus/2(in2)
  fir_tap1/3(c_out) -> outbus_back/15(in15)
  fir_tap1/4(d_out) -> outbus_back/16(in16)
  fir_tap2/1(a_out) -> outbus/3(in3)
  fir_tap2/2(b_out) -> outbus/4(in4)
  fir_tap2/3(c_out) -> outbus_back/13(in13)
  fir_tap2/4(d_out) -> outbus_back/14(in14)
  fir_tap3/1(a_out) -> outbus/5(in5)
  fir_tap3/2(b_out) -> outbus/6(in6)
  fir_tap3/3(c_out) -> outbus_back/11(in11)
  fir_tap3/4(d_out) -> outbus_back/12(in12)
  fir_tap4/1(a_out) -> outbus/7(in7)
  fir_tap4/2(b_out) -> outbus/8(in8)
  fir_tap4/3(c_out) -> outbus_back/9(in9)
  fir_tap4/4(d_out) -> outbus_back/10(in10)
  fir_tap5/1(a_out) -> outbus/9(in9)
  fir_tap5/2(b_out) -> outbus/10(in10)
  fir_tap5/3(c_out) -> outbus_back/7(in7)
  fir_tap5/4(d_out) -> outbus_back/8(in8)
  fir_tap6/1(a_out) -> outbus/11(in11)
  fir_tap6/2(b_out) -> outbus/12(in12)
  fir_tap6/3(c_out) -> outbus_back/5(in5)
  fir_tap6/4(d_out) -> outbus_back/6(in6)
  fir_tap7/1(a_out) -> outbus/13(in13)
  fir_tap7/2(b_out) -> outbus/14(in14)
  fir_tap7/3(c_out) -> outbus_back/3(in3)
  fir_tap7/4(d_out) -> outbus_back/4(in4)
  fir_tap8/1(a_out) -> outbus/15(in15)
  fir_tap8/2(b_out) -> outbus/16(in16)
  fir_tap8/3(c_out) -> outbus_back/1(in1)
  fir_tap8/4(d_out) -> outbus_back/2(in2)
  adder_tree1/1(sync_out) -> term1/1
  adder_tree2/1(sync_out) -> term2/1
  c1/1 -> adder_tree1/1(sync)
  c2/1 -> adder_tree2/1(sync)
  adder_tree1/2(dout) -> real_sum/1
  adder_tree2/2(dout) -> imag_sum/1
  fir_tap1/5(real) -> adder_tree1/2(din1)
  fir_tap1/6(imag) -> adder_tree2/2(din1)
  fir_tap2/5(real) -> adder_tree1/3(din2)
  fir_tap2/6(imag) -> adder_tree2/3(din2)
  fir_tap3/5(real) -> adder_tree1/4(din3)
  fir_tap3/6(imag) -> adder_tree2/4(din3)
  fir_tap4/5(real) -> adder_tree1/5(din4)
  fir_tap4/6(imag) -> adder_tree2/5(din4)
  fir_tap5/5(real) -> adder_tree1/6(din5)
  fir_tap5/6(imag) -> adder_tree2/6(din5)
  fir_tap6/5(real) -> adder_tree1/7(din6)
  fir_tap6/6(imag) -> adder_tree2/7(din6)
  fir_tap7/5(real) -> adder_tree1/8(din7)
  fir_tap7/6(imag) -> adder_tree2/8(din7)
  fir_tap8/5(real) -> adder_tree1/9(din8)
  fir_tap8/6(imag) -> adder_tree2/9(din8)
